simulink model "mass_spring_system_model"  (Simulink 8.1)
settings: Solver=ode45  StartTime=0.0  StopTime=T_end  RelTol=1e-3
values from neighbouring files (symbols this model uses):
  Td = 0.01    [Demo_UE1.m]
undefined symbols (not defined in the file or in its folder): c_id, d_id, m_id, nl
settings Model: Creator=Rumetshofer  LastModifiedBy=Jakob

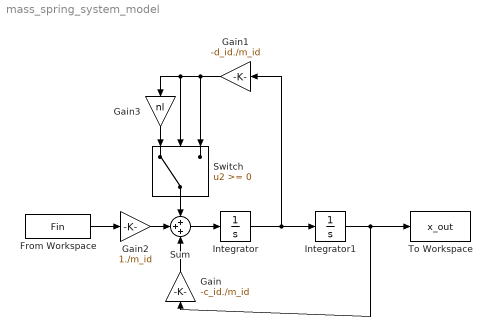
== system mass_spring_system_model ==
  From Workspace : FromWorkspace  VariableName=Fin  SampleTime=Td
  Gain : Gain  Gain=-c_id./m_id
  Gain1 : Gain  Gain=-d_id./m_id
  Gain2 : Gain  Gain=1./m_id
  Gain3 : Gain  Gain=nl
  Integrator : Integrator
  Integrator1 : Integrator
  Sum : Sum  Inputs=+++
  Switch : Switch
  To Workspace : ToWorkspace  VariableName=x_out  SampleTime=Td
  wires:
  Integrator1/1 -> To Workspace/1, Gain/1
  Sum/1 -> Integrator/1
  Gain/1 -> Sum/3
  From Workspace/1 -> Gain2/1
  Gain2/1 -> Sum/2
  Integrator/1 -> Gain1/1, Integrator1/1
  Gain1/1 -> Gain3/1, Switch/2, Switch/3
  Gain3/1 -> Switch/1
  Switch/1 -> Sum/1
